simulink model "Zustandsregelung"  (R2019a)
settings: Solver=VariableStepAuto  StartTime=0.0  StopTime=10.0  RelTol=1e-3
values from neighbouring files (symbols this model uses):
  A = [0 1 0 0;m*g*l(M+m)/d 0 0 m*l*b/d;0 0 0 1;-g*m^2*l^2/d 0 0 -b*(I+m*l^2)/d]    [inv_pend.m]
  B = [0;-m*l/d;0;(I+m*l^2)/d]    [inv_pend.m]
  C = [0 0 1 0;1 0 0 0]    [inv_pend.m]
  K = acker(A,B,5*[-1 -0.5 -0.4 -0.3])    [inv_pend.m]
  V = 1/dcgain(ss(A-B*K,B,Cn,Dn))    [inv_pend.m]
settings Model: Creator=Naveen  LastModifiedBy=Naveen

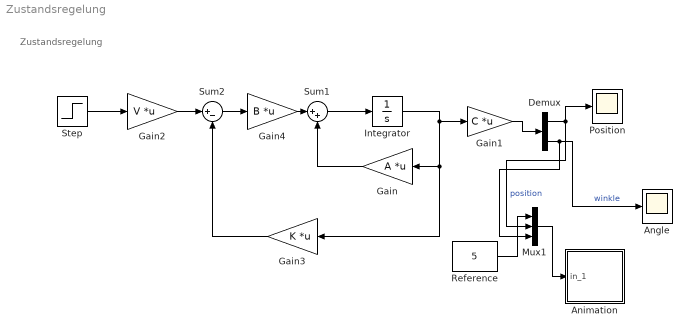
== system Zustandsregelung ==
  note: Zustandsregelung
  Angle : Scope
  Animation : Subsystem  mask(Pendulum plot){RefBlock=Reference}
      mask prompts: RefBlock "DC reference signal block name:"
      mask help: Pendulum plot
      mask Help: Pendulum animation function using Handle graphics.
      mask Display: plot([-10 10],[0 0],[-2 -2 2 2],[0 1 1 0],[0 3],[1 5])
  Demux : Demux  Outputs=2
  Gain : Gain  Gain=A  Multiplication=Matrix(K*u)
  Gain1 : Gain  Gain=C  Multiplication=Matrix(K*u)
  Gain2 : Gain  Gain=V  Multiplication=Matrix(K*u)
  Gain3 : Gain  Gain=K  Multiplication=Matrix(K*u)
  Gain4 : Gain  Gain=B  Multiplication=Matrix(K*u)
  Integrator : Integrator
  Mux1 : Mux  Inputs=3
  Position : Scope
  Reference : Constant  Value=5
  Step : Step  Time=0  After=5  SampleTime=0
  Sum1 : Sum  Inputs=|++
  Sum2 : Sum  Inputs=|+-
  wires:
  Gain4/1 -> Sum1/1
  Gain1/1 -> Demux/1
  Gain2/1 -> Sum2/1
  Step/1 -> Gain2/1
  Sum1/1 -> Integrator/1
  Sum2/1 -> Gain4/1
  Gain/1 -> Sum1/2
  Gain3/1 -> Sum2/2
  Integrator/1 -> Gain1/1, Gain3/1, Gain/1
  Reference/1 -> Mux1/1
  Demux/2 -> Mux1/3, Angle/1  "winkle"
  Mux1/1 -> Animation/1(in_1)
  Demux/1 -> Mux1/2, Position/1  "position"

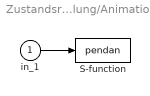
== system Zustandsregelung/Animation ==
  in_1 : Inport
  S-function : S-Function  FunctionName=pendan  Parameters=RefBlock  SFunctionDeploymentMode=off  EnableBusSupport=off
      settings: DeleteFcn=pendan([],[],[],'DeleteBlock');
  wires:
  in_1/1 -> S-function/1
